simulink model "F16_Simulink_Controle_Longitudinal"  (R2013b)
settings: Solver=ode4  StartTime=0.0  StopTime=10  FixedStep=0.01  RelTol=1e-3
InitFcn:
  | close all; clear; clc;
  | 
  | % Carrega as pastas do sistema
  | MainPath = pwd;
  | Folders = {'Turbina'; 'Atmosfera'; 'Modelo';
  |                  'CoeficientesAerodinamicos'};
  | 
  | for i = 1:numel(Folders)
  |     Pasta = [MainPath '/' Folders{i}];
  |     rmpath(Pasta);
  |     addpath(Pasta);
  | end
  | 
  | % Carrega os valores trimados.
  | load('Trimados.mat');
  | 
  | load('Kp.mat');
  | load('Kd.mat');
  | 
  | x0 = x;
  | dt = 0.01;
values from neighbouring files (symbols this model uses):
  x = lat(i)    [DesacopladorDinamicas_Longitudinal_Lateral.m]    (also in Paper_Estudo_Estabilidade.m = vetor(i); Trimados.mat = [502 0.24860688281 -0.00209811994296 1.36614062364 0.0494318; VerificaModeloMatematicoLewis.m = [500 0.5 -0.2 -1 1 -1 0.7 -0.8 0.9 1000 900 10000 90])
settings Model: Creator=Eduardo  LastModifiedBy=Eduardo

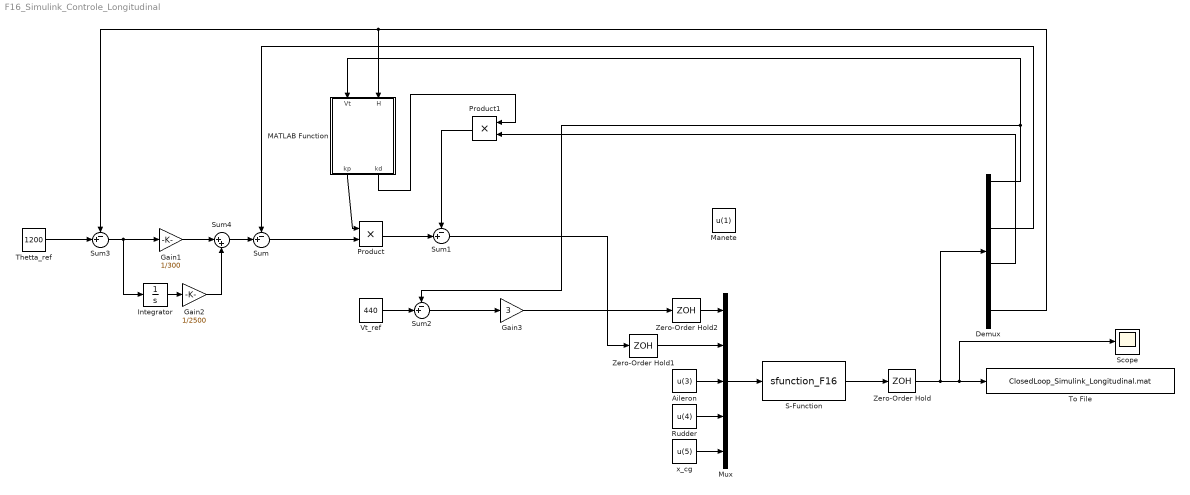
== system F16_Simulink_Controle_Longitudinal ==
  Aileron : Constant  Value=u(3)
  Demux : Demux  Outputs=13
  Gain1 : Gain  Gain=1/300
  Gain2 : Gain  Gain=1/2500
  Gain3 : Gain  Gain=3
  Integrator : Integrator
  MATLAB Function : MATLAB Function  TreatAsAtomicUnit=on
  Manete : Constant  Value=u(1)
  Mux : Mux  Inputs=5
  Product : Product
  Product1 : Product
  Rudder : Constant  Value=u(4)
  S-Function : S-Function  FunctionName=sfunction_F16  Parameters=x0  EnableBusSupport=off
  Scope : Scope
      settings: YMin=-250  YMax=4250
  Sum{,1..3} (4 alike) : Sum  Inputs=-+|
  Sum4 : Sum  Inputs=|++
  Thetta_ref : Constant  Value=1200
  To File : ToFile  Filename=ClosedLoop_Simulink_Longitudinal.mat  SampleTime=0.01
  Vt_ref : Constant  Value=440
  Zero-Order Hold : ZeroOrderHold  SampleTime=dt
  Zero-Order Hold1 : ZeroOrderHold  SampleTime=dt
  Zero-Order Hold2 : ZeroOrderHold  SampleTime=dt
  x_cg : Constant  Value=u(5)
  wires:
  S-Function/1 -> Zero-Order Hold/1
  Rudder/1 -> Mux/4
  Aileron/1 -> Mux/3
  x_cg/1 -> Mux/5
  Mux/1 -> S-Function/1
  Demux/5 -> Sum/1
  Demux/1 -> Sum2/1, MATLAB Function/1(Vt)
  Demux/12 -> MATLAB Function/2(H), Sum3/1
  Zero-Order Hold/1 -> Scope/1, To File/1, Demux/1
  MATLAB Function/1(kp) -> Product/1
  Product/1 -> Sum1/2
  Zero-Order Hold1/1 -> Mux/2
  Demux/8 -> Product1/2
  MATLAB Function/2(kd) -> Product1/1
  Product1/1 -> Sum1/1
  Sum1/1 -> Zero-Order Hold1/1
  Vt_ref/1 -> Sum2/2
  Zero-Order Hold2/1 -> Mux/1
  Sum/1 -> Product/2
  Thetta_ref/1 -> Sum3/2
  Sum3/1 -> Integrator/1, Gain1/1
  Integrator/1 -> Gain2/1
  Sum4/1 -> Sum/2
  Gain1/1 -> Sum4/1
  Gain2/1 -> Sum4/2
  Sum2/1 -> Gain3/1
  Gain3/1 -> Zero-Order Hold2/1

== matlab function F16_Simulink_Controle_Longitudinal/MATLAB Function ==
  data: kp output; kd output; Vt input; H input
function [kp, kd] = fcn(Vt, H)

Kp = [-50   -50   -50   -50   -50   -50   -50   -50   -50   -50   -50;
      -50   -50   -50   -50   -50   -50   -50   -50   -50   -50   -50;
      -50   -50   -50   -50   -50   -50   -50   -50   -50   -50   -50;
      -50   -50   -50   -50   -50   -50   -50   -50   -50   -50   -50;
      -50   -50   -50   -50   -50   -50   -50   -50   -50   -50   -50;
      -50   -50   -50   -50   -50   -50   -50   -50   -50   -50   -50;
      -50   -50   -50   -50   -50   -50   -50   -50   -50   -50   -50;
      -50   -50   -50   -50   -50   -50   -50   -50   -50   -50   -50;
      -50   -50   -50   -50   -50   -50   -50   -50   -50   -50   -50];
  
Kd  = [ -50.0000  -49.7093  -21.7601  -20.7539  -19.5642  -18.2822  -21.1135  -19.7012  -18.4624  -17.3919  -16.4628;
        -50.0000  -49.8079  -21.8419  -20.8417  -19.6596  -18.3832  -21.2586  -19.8178  -18.5670  -17.4888  -16.5541;
        -50.0000  -23.8542  -21.9235  -20.9294  -19.7548  -18.4774  -21.3813  -19.9338  -18.6713  -17.5920  -16.6511;
        -50.0000  -23.9413  -22.0316  -21.0166  -19.8499  -18.5848  -21.5053  -20.0564  -18.7843  -17.6909  -16.7426;
        -50.0000  -24.0278  -22.1114  -21.1061  -19.9448  -18.6856  -21.6212  -20.1667  -18.8945  -17.7940  -16.8375;
        -50.0000  -50.0000  -22.1709  -21.1782  -20.0304  -18.7800  -21.7502  -20.2880  -19.0049  -17.8966  -16.9321;
        -50.0000  -50.0000  -22.2762  -21.2641  -20.1342  -18.8788  -21.8793  -20.4059  -19.1191  -17.9992  -17.0252;
        -50.0000  -50.0000  -22.3598  -21.3662  -21.0837  -18.9792  -22.0050  -20.5236  -19.2316  -18.1052  -17.1261;
        -50.0000  -50.0000  -22.4197  -21.4389  -21.1824  -19.0821  -22.1309  -20.6425  -19.3448  -18.2075  -17.2247];


[kp, kd] = CoeficientesControladores_Interpolados(Kp, Kd, 440, 1200);
